simulink model "temp"  (Simulink 7.7)
settings: Solver=VariableStepDiscrete  SolverMode=SingleTasking  StartTime=0.0  StopTime=50  RelTol=1e-3
model workspace (MATLAB code in the model file):
  | commdvbt_tablegen
undefined symbols (not defined in the file or in its folder): EbNodB, figposition, Fs, gray, M, rsgenpoly, sided, Two
libraries: commblkintrlv2 x6, commutil2 x6, commsink2 x3, dspsigops x3, commblkcod2 x2, commcnvcod2 x2, dspxfrm3 x2, commcnvintrlv2 x2, vipsnks x2, commchan3 x1, commdigbbndam3 x1, vipsrcs x1
Description:
  | Digital Video Broadcasting - Terrestrial
CloseFcn:
  | % Clear global variables
  | clear global GF_TABLE1 GF_TABLE2 GF_TABLE_M GF_TABLE_PRIM_POLY
  | 
  | % Clear signal logging variable
  | clear dvbSigsOut
settings Model: Creator=The MathWorks Inc.  LastModifiedBy=katsikas  ExtModeTrigMode=oneshot  ExtModeArmWhenConnect=off  ExtModeAutoUpdateStatusClock=off  BufferReuse=off
settings SolverCC: ZeroCrossControl=DisableAll
settings DataIOCC: LimitDataPoints=off  SaveOutput=off  SaveTime=off  SignalLoggingName=dvbSigsOut
settings OptimizationCC: BlockReduction=off  BooleanDataType=off  OptimizeBlockIOStorage=off  BufferReuse=off  ExpressionFolding=off  LocalBlockOutputs=off  InitFltsAndDblsToZero=on  EfficientMapNaN2IntZero=off  OptimizeModelRefInitCode=on  LifeSpan=1  BufferReusableBoundary=off
settings DebuggingCC: SaveWithParameterizedLinksMsg=none  CheckExecutionContextPreStartOutputMsg=on  CheckExecutionContextRuntimeOutputMsg=on  SignalResolutionControl=TryResolveAllWithWarning  SolverPrmCheckMsg=none  InheritedTsInSrcMsg=none  MultiTaskDSMMsg=warning  MultiTaskCondExecSysMsg=none  SigSpecEnsureSampleTimeMsg=none  BusObjectLabelMismatch=none  StrictBusMsg=None
settings HardwareCC: TargetBitPerLong=64  TargetBitPerPointer=64  TargetEndianess=LittleEndian  TargetWordSize=64  TargetHWDeviceType=MATLAB Host
settings ModelReferenceCC: UpdateModelReferenceTargets=IfOutOfDate
settings RTWCC: SystemTargetFile=ert.tlc  TemplateMakefile=ert_default_tmf  Description=Real-Time Workshop Embedded Coder (no auto configuration)  RetainRTWFile=on  ProcessScript=ert_make_rtw_hook  IncludeERTFirstTime=on
settings CodeAppCC: IgnoreCustomStorageClasses=off
settings ERTTargetCC: TargetFcnLib=ansi_tfl_tmw.mat  FunctionExecutionProfile=off  MultiwordLength=2048  GenerateSampleERTMain=on  MatFileLogging=on  InlinedParameterPlacement=NonHierarchical  ERTCustomFileTemplate=example_file_process.tlc  ConvertIfToSwitch=off

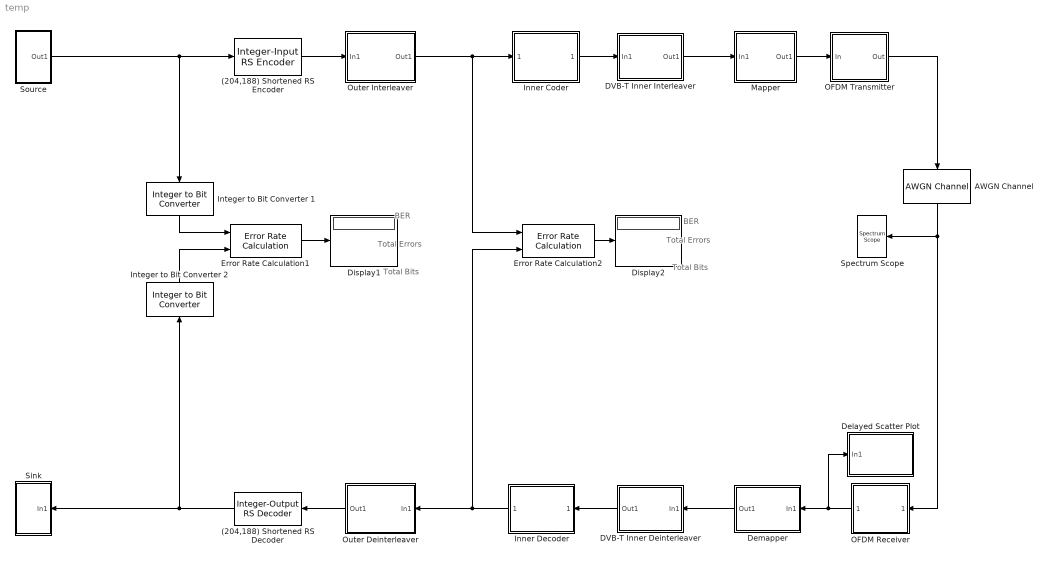
== system temp ==
  note: BER
  note: Total Errors
  note: Total Bits
  note: Total Errors
  note: Total Bits
  note: BER
  (204,188) Shortened RS Decoder : commblkcod2/Integer-Output RS Decoder  n=204  k=188  specPrimPoly=off  prPoly=[1 0 1 1]  specGenPoly=off  genPoly=rsgenpoly(7,3)  specPuncture=off  punctVec=[ones(2,1); zeros(2,1)]  specErasurePort=off  showNumErr=off
  (204,188) Shortened RS Encoder : commblkcod2/Integer-Input RS Encoder  n=204  k=188  specPrimPoly=off  prPoly=[1 0 1 1]  specGenPoly=off  genPoly=rsgenpoly(7,3)  specPuncture=off  punctVec=[ones(2,1); zeros(2,1)]
  AWGN Channel : commchan3/AWGN Channel  SystemSampleTime=-1  InputProcessing=Columns as channels (frame based)  seed=54321  noiseMode="Signal to noise ratio  (SNR)"  EbNodB=10  EsNodB=EbNodB+10*log10(log2(M))  SNRdB=18.5  bitsPerSym=1  Ps=1/2048  Tsym=Tsym  variance=10^(-0.1*15)/(2048*2)
  DVB-T Inner Deinterleaver : Subsystem  mask(DVB-T Inner Deinterleaver){}
      mask init:
      | fullILVec = [(1:126) ...
      |  (rem([0:125]+63,126) +1 + 126     ) ...
      |  (rem([0:125]+105,126)+1 + (2*126) ) ...
      |  (rem([0:125]+42,126) +1 + (3*126) ) ...
      |  (rem([0:125]+21,126) +1 + (4*126) ) ...
      |  (rem([0:125]+84,126) +1 + (5*126) )];
      mask Display: disp('DVB-T\nInner\nDeinterleaver')
  DVB-T Inner Interleaver : Subsystem  mask(DVB-T Inner Interleaver){}
      mask init: same as temp/DVB-T Inner Deinterleaver
      mask Display: disp('DVB-T\nInner\nInterleaver')
  Delayed Scatter Plot : Subsystem
      mask Display: disp('Delayed\nScatter Plot');
  Demapper : Subsystem
      mask Type: DVB-T 64-QAM Demapper
      mask Display: disp('DVB-T\n64-QAM\nDemapper')
  Display1 : Display
  Display2 : Display
  Error Rate Calculation1 : commsink2/Error Rate Calculation  N=188*17*8  st_delay=0  cp_mode=Entire frame  subframe=[]  PMode=Port  WsName=e2  RsMode2=off  stop=on  numErr=100  maxBits=68274180 *8
  Error Rate Calculation2 : commsink2/Error Rate Calculation  N=1632*6  st_delay=0  cp_mode=Entire frame  subframe=[]  PMode=Port  WsName=e1  RsMode2=off  stop=off  numErr=100  maxBits=1e6
  Inner Coder : Subsystem
      mask Display: disp('Rate 3/4\nPunctured\nConvolutional\nCode');
  Inner Decoder : Subsystem
      mask Display: disp('Viterbi\nDecoder')
  Integer to Bit Converter 1 : commutil2/Integer to Bit Converter  nbits=8  signedInputValues=Unsigned  bitOrder=MSB first  outDtype=boolean
  Integer to Bit Converter 2 : commutil2/Integer to Bit Converter  nbits=8  signedInputValues=Unsigned  bitOrder=MSB first  outDtype=boolean
  Mapper : Subsystem
      mask Type: DVB-T 64-QAM Mapper
      mask Display: disp('DVB-T\n64-QAM\nMapper')
  OFDM Receiver : Subsystem
      mask Display: disp('OFDM\nReceiver')
  OFDM Transmitter : Subsystem
      mask Display: disp('OFDM\nTransmitter')
  Outer Deinterleaver : Subsystem
      mask Display: disp('Convolutional\nDeinterleaver\nI=12')
  Outer Interleaver : Subsystem
      mask Display: disp('Convolutional\nInterleaver\nI=12')
  Sink : Subsystem
  Source : Subsystem
  Spectrum Scope : dspsnks4/Spectrum Scope  SystemSampleTime=-1  ScopeProperties=off  Domain=Frequency  HorizSpan=1  UseBuffer=off  BufferSize=128  Overlap=64  TreatMby1Signals=One channel  inpFftLenInherit=off  FFTlength=128  numAvg=2  DisplayProperties=on  AxisGrid=on  Memory=off  FrameNumber=off  AxisLegend=off  AxisZoom=off  OpenScopeAtSimStart=on  OpenScopeImmediately=off  FigPos=figposition([1 7 36 45])  AxisProperties=off  XUnits=Hertz  XRange=Two-sided ((-Fs/2...Fs/2])  XDisplay=0  InheritXIncr=on  XIncr=1.0  XLabel=Samples  XLimit=Auto  YUnits=dBW/Hertz  XMax=1  XMin=0  YLabel=Power spectral density, dBW/Hz  LineProperties=off  wintypeSpecScope=Hann  RsSpecScope=50  betaSpecScope=5  winsampSpecScope=Periodic  XAxisParamsVer=6.9  isFrameUpgraded=on
      settings: YMin=-140  YMax=-90
  wires:
  Source/1(Out1) -> (204,188) Shortened RS Encoder/1, Integer to Bit Converter 1/1
  Mapper/1(Out1) -> OFDM Transmitter/1(In)
  (204,188) Shortened RS Encoder/1 -> Outer Interleaver/1(In1)
  Outer Interleaver/1(Out1) -> Error Rate Calculation2/1, Inner Coder/1(Uncoded symbols)
  OFDM Transmitter/1(Out) -> AWGN Channel/1
  OFDM Receiver/1(OFDM Spectrum) -> Demapper/1(In1), Delayed Scatter Plot/1(In1)
  DVB-T Inner Deinterleaver/1(Out1) -> Inner Decoder/1(Received bits)
  Inner Decoder/1(Decoded symbols) -> Outer Deinterleaver/1(In1), Error Rate Calculation2/2
  Outer Deinterleaver/1(Out1) -> (204,188) Shortened RS Decoder/1
  Error Rate Calculation1/1 -> Display1/1
  Error Rate Calculation2/1 -> Display2/1
  Integer to Bit Converter 2/1 -> Error Rate Calculation1/2
  Integer to Bit Converter 1/1 -> Error Rate Calculation1/1
  DVB-T Inner Interleaver/1(Out1) -> Mapper/1(In1)
  Inner Coder/1(Coded bits) -> DVB-T Inner Interleaver/1(In1)
  Demapper/1(Out1) -> DVB-T Inner Deinterleaver/1(In1)
  AWGN Channel/1 -> OFDM Receiver/1(Received signal), Spectrum Scope/1
  (204,188) Shortened RS Decoder/1 -> Sink/1(In1), Integer to Bit Converter 2/1

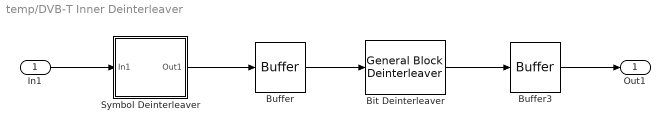
== system temp/DVB-T Inner Deinterleaver ==
  In1 : Inport
  Bit Deinterleaver : commblkintrlv2/General Block Deinterleaver  elements=dvb_bit_int_table
  Buffer : Buffer  N=756  TreatMby1Signals=One channel
  Buffer3 : Buffer  N=2176  TreatMby1Signals=One channel
  Symbol Deinterleaver : Subsystem
      mask Display:
      | port_label('input', 1, '')
      | port_label('output', 1, '')
      | disp('Symbol\nDeinterleaver')
  Out1 : Outport
  wires:
  Buffer/1 -> Bit Deinterleaver/1
  In1/1 -> Symbol Deinterleaver/1(In1)
  Bit Deinterleaver/1 -> Buffer3/1
  Buffer3/1 -> Out1/1
  Symbol Deinterleaver/1(Out1) -> Buffer/1

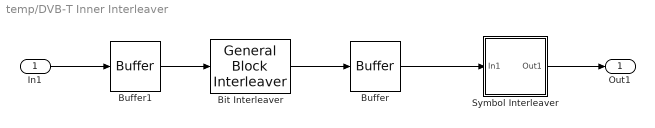
== system temp/DVB-T Inner Interleaver ==
  In1 : Inport
  Bit Interleaver : commblkintrlv2/General Block Interleaver  elements=dvb_bit_int_table
  Buffer : Buffer  N=9072  TreatMby1Signals=One channel
  Buffer1 : Buffer  N=756  TreatMby1Signals=One channel
  Symbol Interleaver : Subsystem
      mask Display:
      | port_label('input', 1, '')
      | port_label('output', 1, '')
      | disp('Symbol\nInterleaver')
  Out1 : Outport
  wires:
  Buffer1/1 -> Bit Interleaver/1
  In1/1 -> Buffer1/1
  Bit Interleaver/1 -> Buffer/1
  Symbol Interleaver/1(Out1) -> Out1/1
  Buffer/1 -> Symbol Interleaver/1(In1)

== system temp/Delayed Scatter Plot ==
  In1 : Inport
  Enabled Scatter Plot : Subsystem  TreatAsAtomicUnit=on
  Step : Step  Time=.001  SampleTime=.000224
  wires:
  Step/1 -> Enabled Scatter Plot/Enable
  In1/1 -> Enabled Scatter Plot/1(In1)

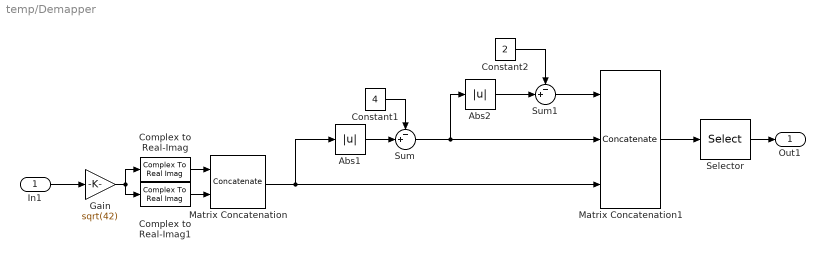
== system temp/Demapper ==
  In1 : Inport
  Abs1 : Abs  SaturateOnIntegerOverflow=on
  Abs2 : Abs  SaturateOnIntegerOverflow=on
  Complex to Real-Imag : ComplexToRealImag  Output=Imag
  Complex to Real-Imag1 : ComplexToRealImag  Output=Real
  Constant1 : Constant  Value=4
  Constant2 : Constant  Value=2
  Gain : Gain  Gain=sqrt(42)  SaturateOnIntegerOverflow=on  OutDataTypeStr=Inherit: Same as input  ParamDataTypeStr=Inherit: Same as input
  Matrix Concatenation : Concatenate  Mode=Multidimensional array
  Matrix Concatenation1 : Concatenate  NumInputs=3  Mode=Multidimensional array
  Selector : Selector  NumberOfDimensions=2  InputPortWidth=9072  IndexOptions=Index vector (dialog),Select all  Indices=reshape(reshape(1:9072,1512,6)',9072,1),1  OutputSizes=1,1
  Sum : Sum  Inputs=-+|  SaturateOnIntegerOverflow=on  InputSameDT=on  OutDataTypeStr=Inherit: Same as first input
  Sum1 : Sum  Inputs=-+|  SaturateOnIntegerOverflow=on  InputSameDT=on  OutDataTypeStr=Inherit: Same as first input
  Out1 : Outport
  wires:
  Matrix Concatenation/1 -> Abs1/1, Matrix Concatenation1/3
  Gain/1 -> Complex to Real-Imag/1, Complex to Real-Imag1/1
  Complex to Real-Imag1/1 -> Matrix Concatenation/2
  Complex to Real-Imag/1 -> Matrix Concatenation/1
  Sum/1 -> Abs2/1, Matrix Concatenation1/2
  Abs1/1 -> Sum/2
  Constant1/1 -> Sum/1
  Constant2/1 -> Sum1/1
  Abs2/1 -> Sum1/2
  Selector/1 -> Out1/1
  Sum1/1 -> Matrix Concatenation1/1
  In1/1 -> Gain/1
  Matrix Concatenation1/1 -> Selector/1

== system temp/Inner Coder ==
  Uncoded symbols : Inport
  Convolutional  Encoder : commcnvcod2/Convolutional Encoder  trellis=poly2trellis(7, [171 133])  opMode=Continuous  DelayedResetAction=off  hasIniStPort=off  hasFinStPort=off  usePuncVector=on  punctureVector=[1 1 0 1 1 0]'  reset=Unused parameter value
  Coded bits : Outport
  wires:
  Convolutional  Encoder/1 -> Coded bits/1
  Uncoded symbols/1 -> Convolutional  Encoder/1

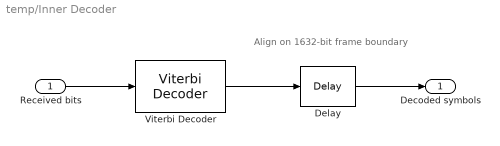
== system temp/Inner Decoder ==
  note: Align on 1632-bit
      | frame boundary
  Received bits : Inport
  Delay : dspsigops/Delay  InputProcessing=Columns as channels (frame based)  dly_unit=Samples  delay=584+69  ic_detail=off  dif_ic_for_ch=off  dif_ic_for_dly=off  ic=0  reset_popup=None
  Viterbi Decoder : commcnvcod2/Viterbi Decoder  trellis=poly2trellis(7, [171 133])  isPunctured=on  punctureVector=[1 1 0 1 1 0]'  erasures=off  dectype=Unquantized  runSigValErrCheck=off  nsdecb=4  smWordLength=16  tbdepth=136  opmode=Continuous  reset=off  outDataType=boolean
  Decoded symbols : Outport
  wires:
  Viterbi Decoder/1 -> Delay/1
  Received bits/1 -> Viterbi Decoder/1
  Delay/1 -> Decoded symbols/1

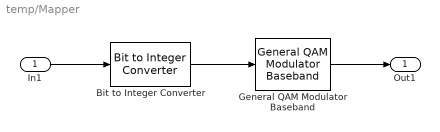
== system temp/Mapper ==
  In1 : Inport
  Bit to Integer Converter : commutil2/Bit to Integer Converter  nbits=6  bitOrder=MSB first  signedOutputValues=Unsigned  outDtype=uint8  outDtypeSigned=Inherit via internal rule
  General QAM Modulator Baseband : commdigbbndam3/General QAM Modulator Baseband  SigCon=dvbt_qam  outDtype=double  outWordLen=16  outUDDataType=sfix(16)  outFracLenMode=Best precision  outFracLen=15
  Out1 : Outport
  wires:
  General QAM Modulator Baseband/1 -> Out1/1
  In1/1 -> Bit to Integer Converter/1
  Bit to Integer Converter/1 -> General QAM Modulator Baseband/1

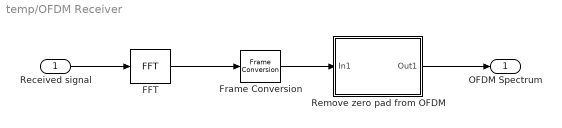
== system temp/OFDM Receiver ==
  Received signal : Inport
  FFT : dspxfrm3/FFT  CompMethod=Table lookup  TableOpt=NEW  TableOptActive=Speed  BitRevOrder=off  InheritFFTLength=on  FFTLength=64  RowConvenienceOn=on  SkipNorm=off  firstCoeffMode=Specify word length  firstCoeffWordLength=16  firstCoeffFracLength=15  firstCoeffDataTypeStr=fixdt(1,16)  firstCoeffLastDataTypeStr=fixdt(1,16)  outputMin=[]  outputMax=[]  accumDataTypeStr=Inherit: Same as product output  accumLastDataTypeStr=Inherit: Same as product output  roundingMode=Floor  overflowMode=off
  Frame Conversion : FrameConversion
  Remove zero pad from OFDM : Subsystem
      mask Display: disp('Remove zero\npad from OFDM');
  OFDM Spectrum : Outport
  wires:
  Remove zero pad from OFDM/1(Out1) -> OFDM Spectrum/1
  Received signal/1 -> FFT/1
  FFT/1 -> Frame Conversion/1
  Frame Conversion/1 -> Remove zero pad from OFDM/1(In1)

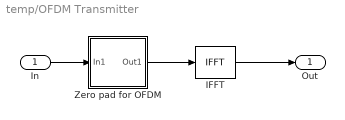
== system temp/OFDM Transmitter ==
  In : Inport
  IFFT : dspxfrm3/IFFT  CompMethod=Table lookup  TableOpt=HYBRID  TableOptActive=Speed  BitRevOrder=off  cs_in=off  SkipNorm=on  InheritFFTLength=on  FFTLength=64  mode=Complex  outSamplingMode=Frame based  RowConvenienceOn=on  firstCoeffMode=User-defined  firstCoeffWordLength=16  firstCoeffFracLength=15  firstCoeffDataTypeStr=fixdt(1,16)  firstCoeffLastDataTypeStr=fixdt(1,16)  outputMin=[]  outputMax=[]  accumDataTypeStr=Inherit: Same as product output  accumLastDataTypeStr=Inherit: Same as product output  roundingMode=Floor  overflowMode=off
  Zero pad for OFDM : Subsystem
      mask Display: disp('Zero pad\nfor OFDM');
  Out : Outport
  wires:
  IFFT/1 -> Out/1
  In/1 -> Zero pad for OFDM/1(In1)
  Zero pad for OFDM/1(Out1) -> IFFT/1

== system temp/Outer Deinterleaver ==
  In1 : Inport
  Bit to Integer Converter : commutil2/Bit to Integer Converter  nbits=8  bitOrder=MSB first  signedOutputValues=Unsigned  outDtype=uint8  outDtypeSigned=Inherit via internal rule
  Convolutional Deinterleaver : commcnvintrlv2/Convolutional Deinterleaver  SystemSampleTime=-1  N=12  B=17  ic=0
  Out1 : Outport
  wires:
  In1/1 -> Bit to Integer Converter/1
  Convolutional Deinterleaver/1 -> Out1/1
  Bit to Integer Converter/1 -> Convolutional Deinterleaver/1

== system temp/Outer Interleaver ==
  In1 : Inport
  Convolutional Interleaver : commcnvintrlv2/Convolutional Interleaver  SystemSampleTime=-1  N=12  B=17  ic=0
  Integer to Bit Converter : commutil2/Integer to Bit Converter  nbits=8  signedInputValues=Unsigned  bitOrder=MSB first  outDtype=boolean
  Out1 : Outport
  wires:
  Integer to Bit Converter/1 -> Out1/1
  Convolutional Interleaver/1 -> Integer to Bit Converter/1
  In1/1 -> Convolutional Interleaver/1

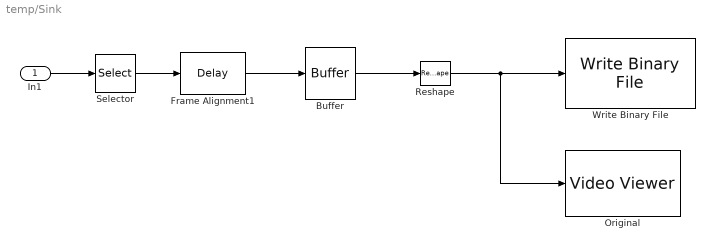
== system temp/Sink ==
  In1 : Inport
  Buffer : Buffer  N=512*736  TreatMby1Signals=One channel
  Frame Alignment1 : dspsigops/Delay  InputProcessing=Columns as channels (frame based)  dly_unit=Samples  delay=(512*736*2) - 379960  ic_detail=off  dif_ic_for_ch=off  dif_ic_for_dly=off  ic=0  reset_popup=None
  Original : vipsnks/Video Viewer  inputType=Obsolete7b  imagePorts=One multidimensional signal  useColorMap=off  colormapValue=gray(256)  specRange=off  minInputVal=0  maxInputVal=255  FigPos=[97 966 410 300]  AxisZoom=on  trueSizedOnce=on  OpenAtMdlStart=on
  Reshape : Reshape  OutputDimensionality=Customize  OutputDimensions=[512,736]
  Selector : Selector  NumberOfDimensions=2  InputPortWidth=1  IndexOptions=Index vector (dialog),Index vector (dialog)  Indices=[5:188],1  OutputSizes=1,1
  Write Binary File : vipsnks/Write Binary File  FileName=example.ts  VideoFormat=Custom  FOURCC=I420  BitStreamFormat=Planar  NumInputs=1  ComponentOrder=[1]  Interlaced=off  LineOrdering=Top line first  InheritBits=off  Component1=Y'  Component2=Cb  Component3=Cr  Component4=Alpha  Bits1=8  Bits2=8  Bits3=8  Bits4=0  SignedInput=off  FileEndian=Little endian
  wires:
  In1/1 -> Selector/1
  Reshape/1 -> Original/1, Write Binary File/1
  Buffer/1 -> Reshape/1
  Selector/1 -> Frame Alignment1/1
  Frame Alignment1/1 -> Buffer/1

== system temp/Source ==
  MPEG2 Source : Subsystem
  MPEG2 TS : Subsystem
  Out1 : Outport
  wires:
  MPEG2 Source/1(Out1) -> MPEG2 TS/1(In1)
  MPEG2 TS/1(MPEG-2 Trnsp) -> Out1/1

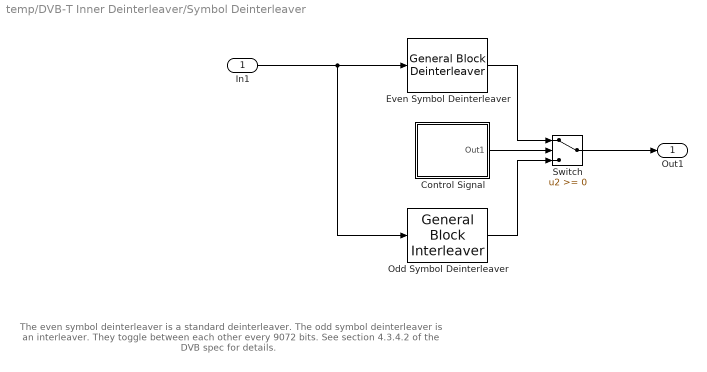
== system temp/DVB-T Inner Deinterleaver/Symbol Deinterleaver ==
  note: The even symbol deinterleaver is a standard deinterleaver.  The odd symbol deinterleaver is an interleaver.  They toggle
      | between each other every 9072 bits.  See section 4.3.4.2 of the DVB spec for details.
  In1 : Inport
  Control Signal : Subsystem
      mask Display:
      | port_label('output', 1, 'ctrl')
      | disp('Control\nSignal')
  Even Symbol Deinterleaver : commblkintrlv2/General Block Deinterleaver  elements=dvb_sym_int_table
  Odd Symbol Deinterleaver : commblkintrlv2/General Block Interleaver  elements=dvb_sym_int_table
  Switch : Switch
  Out1 : Outport
  wires:
  In1/1 -> Odd Symbol Deinterleaver/1, Even Symbol Deinterleaver/1
  Switch/1 -> Out1/1
  Control Signal/1(Out1) -> Switch/2
  Even Symbol Deinterleaver/1 -> Switch/1
  Odd Symbol Deinterleaver/1 -> Switch/3

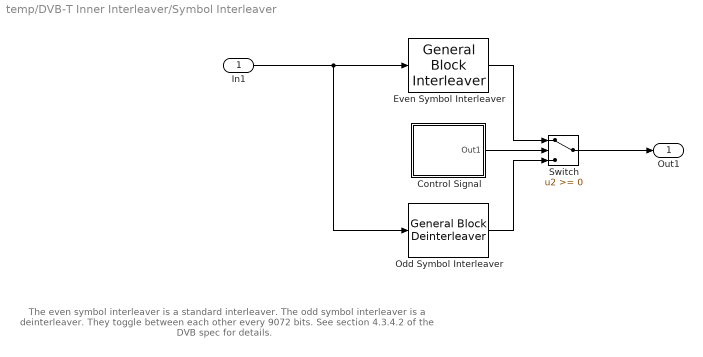
== system temp/DVB-T Inner Interleaver/Symbol Interleaver ==
  note: The even symbol interleaver is a standard interleaver.  The odd symbol interleaver is a deinterleaver.  They toggle
      | between each other every 9072 bits.  See section 4.3.4.2 of the DVB spec for details.
  In1 : Inport
  Control Signal : Subsystem
      mask Display:
      | port_label('output', 1, 'ctrl')
      | disp('Control\nSignal')
  Even Symbol Interleaver : commblkintrlv2/General Block Interleaver  elements=dvb_sym_int_table
  Odd Symbol Interleaver : commblkintrlv2/General Block Deinterleaver  elements=dvb_sym_int_table
  Switch : Switch
  Out1 : Outport
  wires:
  In1/1 -> Even Symbol Interleaver/1, Odd Symbol Interleaver/1
  Switch/1 -> Out1/1
  Control Signal/1(Out1) -> Switch/2
  Even Symbol Interleaver/1 -> Switch/1
  Odd Symbol Interleaver/1 -> Switch/3

== system temp/Delayed Scatter Plot/Enabled Scatter Plot ==
  In1 : Inport
  Enable : EnablePort  PropagateVarSize=During execution
  Discrete-Time Scatter Plot Scope : commsink2/Discrete-Time Scatter Plot Scope  Tag=ScatterPlot  SystemSampleTime=-1  sampPerSymb=1  offsetEye=0  numTraces=1512*3  numNewFrames=1512  LineMarkers=.  LineColors=b  fading=off  render=off  AxisGrid=on  xMin=-1.57132687953875  xMax=1.56234519882275  yMin=-1.59183645307302  yMax=1.54183562528848  inphaseLabel=In-phase Amplitude  quadratureLabel=Quadrature Amplitude  openScopeAtSimStart=on  FrameNumber=off  FigPos=figposition([64 7 35 47])  figTitle=Signal from OFDM Receiver  numLinesMax=50  block_type_=scatter
  wires:
  In1/1 -> Discrete-Time Scatter Plot Scope/1

== system temp/OFDM Receiver/Remove zero pad from OFDM ==
  In1 : Inport
  Selector : Selector  NumberOfDimensions=2  InputPortWidth=2048  IndexOptions=Index vector (dialog),Select all  Indices=[1:756 1293:2048],1  OutputSizes=1,1
  Out1 : Outport
  wires:
  In1/1 -> Selector/1
  Selector/1 -> Out1/1

== system temp/OFDM Transmitter/Zero pad for OFDM ==
  In1 : Inport
  Selector : Selector  NumberOfDimensions=2  InputPortWidth=2048  IndexOptions=Index vector (dialog),Select all  Indices="[1:756 1513:2048  757:1512],1"  OutputSizes=1,1
  Zero Pad : dspsigops/Pad  padAlong=Columns  dimsToPad=1  valSrc=Specify via dialog  padVal=0  spec=Output size  padNumOutRowsSpecMethod=User-specified  numOutRows=2048  padNumOutColsSpecMethod=User-specified  numOutCols=1  isVarDimsMode=off  padBeginning=0  padEnd=0  outSizeMode=User-specified  outSize=1  padSigAt=End  trunc_flag=None  roundingMode=Floor  overflowMode=off  truncOrWrapMode=Truncate  wrap_flag=None
  Out1 : Outport
  wires:
  In1/1 -> Zero Pad/1
  Selector/1 -> Out1/1
  Zero Pad/1 -> Selector/1

== system temp/Source/MPEG2 Source ==
  Buffer : Buffer  N=184  TreatMby1Signals=One channel
  Read Binary File : vipsrcs/Read Binary File  FileName=/home/katsikas/katsikas-repo/Simulink/Korgialas_GeiaSou.ts  loopOrNot=on  numLoops=1  VideoFormat=Custom  FOURCC=I420  BitStreamFormat=Planar  NumOutputs=1  ComponentOrder=[1]  Interlaced=off  LineOrdering=Top line first  Ts=1/9  Component1=Y'  Component2=Cb  Component3=Cr  Component4=Alpha  Bits1=8  Bits2=8  Bits3=8  Bits4=8  Rows1=512  Rows2=60  Rows3=60  Rows4=288  Cols1=736  Cols2=80  Cols3=80  Cols4=352  YRows=288  YCols=352  SignedOutput=off  FileEndian=Little endian  OutputEOF=off
  Reshape : Reshape  OutputDimensionality=Column vector (2-D)
  Out1 : Outport
  wires:
  Read Binary File/1 -> Reshape/1
  Reshape/1 -> Buffer/1
  Buffer/1 -> Out1/1

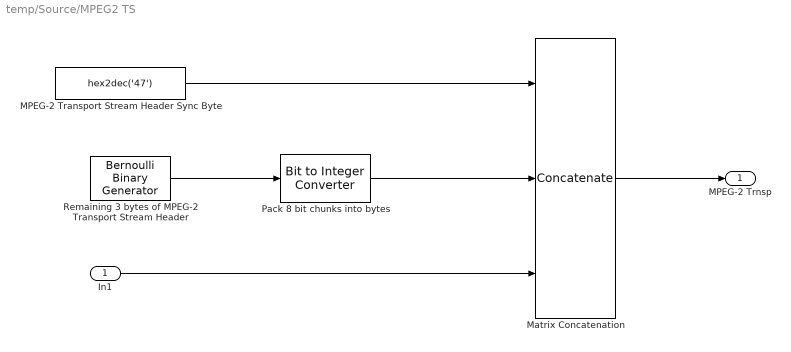
== system temp/Source/MPEG2 TS ==
  In1 : Inport
  MPEG-2 Transport Stream Header Sync Byte : Constant  Value=hex2dec('47')  VectorParams1D=off  OutDataTypeStr=uint8  FramePeriod=8*188/9
      settings: SamplingMode=Frame based
  Matrix Concatenation : Concatenate  NumInputs=3  Mode=Multidimensional array
  Pack 8 bit chunks into bytes : commutil2/Bit to Integer Converter  nbits=8  bitOrder=MSB first  signedOutputValues=Unsigned  outDtype=uint8  outDtypeSigned=Inherit via internal rule
  Remaining 3 bytes of MPEG-2 Transport Stream Header : commrandsrc2/Bernoulli Binary Generator  SystemSampleTime=-1  P=1  seed=61  Ts=(8*188/9) / (3*8)  frameBased=on  sampPerFrame=3*8  orient=off  outDataType=uint8
  MPEG-2 Trnsp : Outport
  wires:
  MPEG-2 Transport Stream Header Sync Byte/1 -> Matrix Concatenation/1
  Remaining 3 bytes of MPEG-2 Transport Stream Header/1 -> Pack 8 bit chunks into bytes/1
  Matrix Concatenation/1 -> MPEG-2 Trnsp/1
  Pack 8 bit chunks into bytes/1 -> Matrix Concatenation/2
  In1/1 -> Matrix Concatenation/3

== system temp/DVB-T Inner Deinterleaver/Symbol Deinterleaver/Control Signal ==
  note: Generate a control signal that toggles between +/- 1 every frame of 9072 bits
  DSP Constant1 : Constant  VectorParams1D=off
  Pulse Generator : DiscretePulseGenerator  Amplitude=2  SampleTime=-1
  Subtract : Sum  Inputs=|+-
  Out1 : Outport
  wires:
  Subtract/1 -> Out1/1
  DSP Constant1/1 -> Subtract/2
  Pulse Generator/1 -> Subtract/1

== system temp/DVB-T Inner Interleaver/Symbol Interleaver/Control Signal ==
  note: Generate a control signal that toggles between +/- 1 every frame of 9072 bits
  DSP Constant1 : Constant  VectorParams1D=off
  Pulse Generator : DiscretePulseGenerator  Amplitude=2  SampleTime=-1
  Subtract : Sum  Inputs=|+-
  Out1 : Outport
  wires:
  Subtract/1 -> Out1/1
  DSP Constant1/1 -> Subtract/2
  Pulse Generator/1 -> Subtract/1
